simulink model "minimalist11_former03"  (Simulink 7.4)
settings: Solver=FixedStepDiscrete  StartTime=0.0  StopTime=inf  FixedStep=0.01  RelTol=1e-3
PreLoadFcn:
  | RTWConfigurationCB('preloadfcn', bdroot);
PostLoadFcn:
  | mpc555rt_switch_target(gcs,'auto')
libraries: mpc555drivers x3
CloseFcn:
  | rtwprivate ssgencode ModelCloseRequest foo
settings Model: Creator=The MathWorks Inc.  LastModifiedBy=autopilot
settings DataIOCC: LimitDataPoints=off  SignalLoggingName=sigsOut
settings OptimizationCC: InlineParams=on  InlineInvariantSignals=on  EnforceIntegerDowncast=off  ZeroExternalMemoryAtStartup=off  ZeroInternalMemoryAtStartup=off  InitFltsAndDblsToZero=on  NoFixptDivByZeroProtection=on  OptimizeModelRefInitCode=on  LifeSpan=1
settings DebuggingCC: SaveWithParameterizedLinksMsg=none  SignalResolutionControl=TryResolveAllWithWarning  SolverPrmCheckMsg=none  MultiTaskDSMMsg=warning  MultiTaskCondExecSysMsg=none  UnderSpecifiedDataTypeMsg=error  StrictBusMsg=None
settings HardwareCC: ProdEndianess=BigEndian  ProdHWDeviceType=Motorola PowerPC
settings RTWCC: SystemTargetFile=mpc555rt.tlc  TemplateMakefile=mpc555rt.tmf  Description=Target Support Package (for use with Freescale MPC5xx) (real-time)  ProcessScript=mpc555rt_make_rtw_hook
settings CodeAppCC: IgnoreCustomStorageClasses=off
settings STFCustomTargetCC: TargetFcnLib=ansi_tfl_tmw.mat  TargetLibSuffix=.a  TargetPreCompLibLocation=C:\Program Files\MATLAB\R2009b\toolbox\rtw\targets\mpc555dk\drivers\lib\DIAB  IncludeMdlTerminateFcn=off  CombineOutputUpdateFcns=on  ERTCustomFileBanners=on  SupportAbsoluteTime=off  SupportNonFinite=off  SupportComplex=off  SupportContinuousTime=off  SupportNonInlinedSFcns=off  CPPClassGenCompliant=on  SystemTargetFile=mpc555rt.tlc
settings ERTTargetCC: TargetFcnLib=ansi_tfl_tmw.mat  TargetPreCompLibLocation=C:\Program Files\MATLAB\R2009b\toolbox\rtw\targets\mpc555dk\drivers\lib\DIAB  MultiwordLength=2048  ParMdlRefBuildCompliant=off  CompOptLevelCompliant=off  IncludeMdlTerminateFcn=off  ERTFirstTimeCompliant=off  SupportAbsoluteTime=off  SupportNonFinite=off  SupportComplex=off  ModelStepFunctionPrototypeControlCompliant=off  ExtModeMexFile=MPC5xxExternalModeOpen  ExtModeIntrfLevel=Level2 - Open  ERTCustomFileTemplate=example_file_process.tlc  ConvertIfToSwitch=off
settings CustomProperty: DataType=RTWOptions_EnumType__toolbox_rtw_targets_mpc555dk_mpc555dk_mpc555rt_1MPC555_OPTIMIZATION_SWITCH  Value=speed
settings EnumStrPairs: String=speed

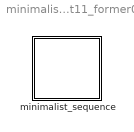
== system minimalist11_former03 ==
  minimalist_sequence : Subsystem  InitFcn=|
      | % START RTW CONFIGURATION CODE %
      | RTWConfigurationCB('rtw_target_initfcn',gcb);
      | % END RTW CONFIGURATION CODE %
      mask Display: image(imread('target_affordance_icon.jpg'),'bottom-right')

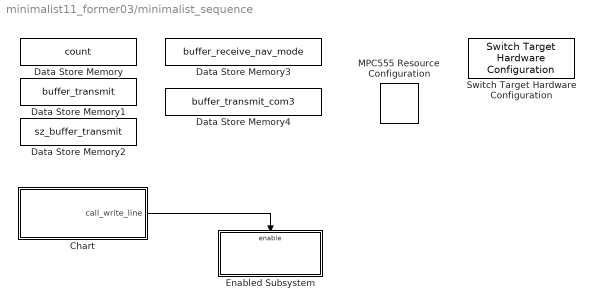
== system minimalist11_former03/minimalist_sequence ==
  Chart : Stateflow chart
  Data Store Memory : DataStoreMemory  DataStoreName=count  DataType=uint8  OutDataType=fixdt(1, 16)  OutScaling=2^0  OutDataTypeStr=uint8
  Data Store Memory1 : DataStoreMemory  DataStoreName=buffer_transmit  InitialValue=[0 0 0 0 0 0 0 0 0 0 0]  DataType=uint8  OutDataType=fixdt(1, 16)  OutScaling=2^0  OutDataTypeStr=uint8
  Data Store Memory2 : DataStoreMemory  DataStoreName=sz_buffer_transmit  DataType=uint32  OutDataType=fixdt(1, 16)  OutScaling=2^0  OutDataTypeStr=uint32
  Data Store Memory3 : DataStoreMemory  DataStoreName=buffer_receive_nav_mode  InitialValue=[0 0 0 0 0 0 0 0 0 0 0 0 0 0 0 0 0 0 0 0 0 0 0 0 0 0 0 0 0 0 0 0 0 0 0 0 0]  DataType=uint8  OutDataType=fixdt(1, 16)  OutScaling=2^0  OutDataTypeStr=uint8
  Data Store Memory4 : DataStoreMemory  DataStoreName=buffer_transmit_com3  InitialValue=[65 66 67 68 69 70 71 72 73 74 75 76 77 78 79 13 10]  DataType=uint8  OutDataType=fixdt(1, 16)  OutScaling=2^0  OutDataTypeStr=uint8
  Enabled Subsystem : Subsystem  TreatAsAtomicUnit=on
  MPC555 Resource Configuration : mpc555drivers/MPC555 Resource Configuration  Tag=RTW CONFIGURATION BLOCK  Priority=-100000  SystemSampleTime=-1  oldParentName=minimalist11_former03/minimalist_sequence  oldBlockName=|
      | minimalist11_former03/minimalist_sequence/MPC555
      | Resource
      | Configuration
  Switch Target Hardware Configuration : mpc555drivers/Utilities/Switch Target Hardware Configuration  SystemSampleTime=-1
  wires:
  Chart/1(call_write_line) -> Enabled Subsystem/Enable

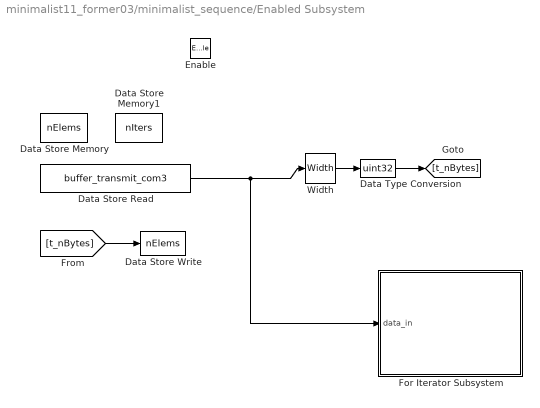
== system minimalist11_former03/minimalist_sequence/Enabled Subsystem ==
  Enable : EnablePort
  Data Store Memory : DataStoreMemory  DataStoreName=nElems  DataType=uint32  OutDataType=fixdt(1, 16)  OutScaling=2^0  OutDataTypeStr=uint32
  Data Store Memory1 : DataStoreMemory  DataStoreName=nIters  DataType=uint32  OutDataType=fixdt(1, 16)  OutScaling=2^0  OutDataTypeStr=uint32
  Data Store Read : DataStoreRead  DataStoreName=buffer_transmit_com3  SampleTime=-1
  Data Store Write : DataStoreWrite  DataStoreName=nElems  SampleTime=-1
  Data Type Conversion : DataTypeConversion  OutDataTypeMode=uint32  OutDataType=fixdt(1, 16)  OutScaling=2^0  OutDataTypeStr=uint32
  For Iterator Subsystem : Subsystem  TreatAsAtomicUnit=on
  Width : Width
  wires:
  Data Store Read/1 -> Width/1, For Iterator Subsystem/1(data_in)
  Width/1 -> Data Type Conversion/1
  Data Type Conversion/1 -> [t_nBytes]
  [t_nBytes] -> Data Store Write/1

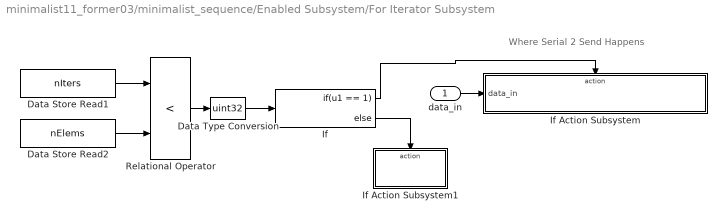
== system minimalist11_former03/minimalist_sequence/Enabled Subsystem/For Iterator Subsystem ==
  note: Where Serial 2 Send Happens
  data_in : Inport  DataType=uint8  OutDataType=fixdt(1, 16)  OutScaling=2^0  OutDataTypeStr=uint8
  Data Store Read1 : DataStoreRead  DataStoreName=nIters  SampleTime=-1
  Data Store Read2 : DataStoreRead  DataStoreName=nElems  SampleTime=-1
  Data Type Conversion : DataTypeConversion  OutDataTypeMode=uint32  OutDataType=fixdt(1, 16)  OutScaling=2^0  OutDataTypeStr=uint32
  If : If  IfExpression=u1 == 1
  If Action Subsystem : Subsystem  TreatAsAtomicUnit=on
  If Action Subsystem1 : Subsystem  TreatAsAtomicUnit=on
  Relational Operator : RelationalOperator  Operator=<  LogicOutDataTypeMode=boolean  LogicDataType=fixdt(0, 8)  OutDataTypeStr=boolean  InputSameDT=on
  wires:
  Data Store Read1/1 -> Relational Operator/1
  Data Store Read2/1 -> Relational Operator/2
  Relational Operator/1 -> Data Type Conversion/1
  Data Type Conversion/1 -> If/1
  If/1 -> If Action Subsystem/Action
  If/2 -> If Action Subsystem1/Action
  data_in/1 -> If Action Subsystem/1(data_in)

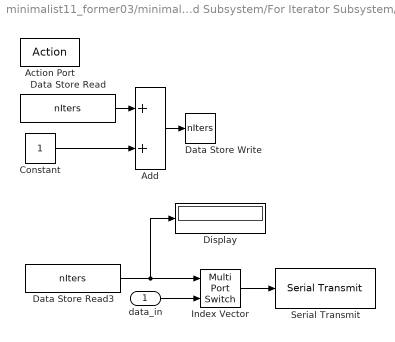
== system minimalist11_former03/minimalist_sequence/Enabled Subsystem/For Iterator Subsystem/If Action Subsystem ==
  data_in : Inport  DataType=uint8  OutDataType=fixdt(1, 16)  OutScaling=2^0  OutDataTypeStr=uint8
  Action Port : ActionPort
  Add : Sum  OutDataType=fixdt(1, 16)  OutScaling=2^-10
  Constant : Constant  OutDataTypeMode=uint32  OutDataType=fixdt(1, 16)  OutScaling=2^0  OutDataTypeStr=uint32
  Data Store Read : DataStoreRead  DataStoreName=nIters  SampleTime=-1
  Data Store Read3 : DataStoreRead  DataStoreName=nIters  SampleTime=-1
  Data Store Write : DataStoreWrite  DataStoreName=nIters  SampleTime=-1
  Display : Display
  Index Vector : MultiPortSwitch  Inputs=1  OutDataType=fixdt(1, 16)  OutScaling=2^0
  Serial Transmit : mpc555drivers/Serial Communications Interface (SCI)/Serial Transmit  module=2  show_length=off  show_num_sent=off  T=-1
  wires:
  Constant/1 -> Add/2
  Data Store Read/1 -> Add/1
  Add/1 -> Data Store Write/1
  Data Store Read3/1 -> Index Vector/1, Display/1
  data_in/1 -> Index Vector/2
  Index Vector/1 -> Serial Transmit/1

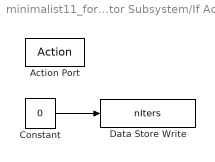
== system minimalist11_former03/minimalist_sequence/Enabled Subsystem/For Iterator Subsystem/If Action Subsystem1 ==
  Action Port : ActionPort
  Constant : Constant  Value=0  OutDataTypeMode=uint32  OutDataType=fixdt(1, 16)  OutScaling=2^0  OutDataTypeStr=uint32
  Data Store Write : DataStoreWrite  DataStoreName=nIters  SampleTime=-1
  wires:
  Constant/1 -> Data Store Write/1

== stateflow chart minimalist_sequence/Chart ==
  state STEP01
    call_write_line=1;
    cnt=cnt+1;
  state END
    call_write_line=0;
  (default) -> STEP01
  STEP01 -> END [order 1] : [cnt>=10]
  STEP01 -> STEP01 [order 2] : [cnt<10]
  data: call_write_line output uint8; cnt local uint8 =0
